simulink model "newmodel"  (R2020b)
settings: Solver=VariableStepAuto  StartTime=0.0  StopTime=10.0  RelTol=1e-3
settings Model: Creator=Obian  LastModifiedBy=Obian

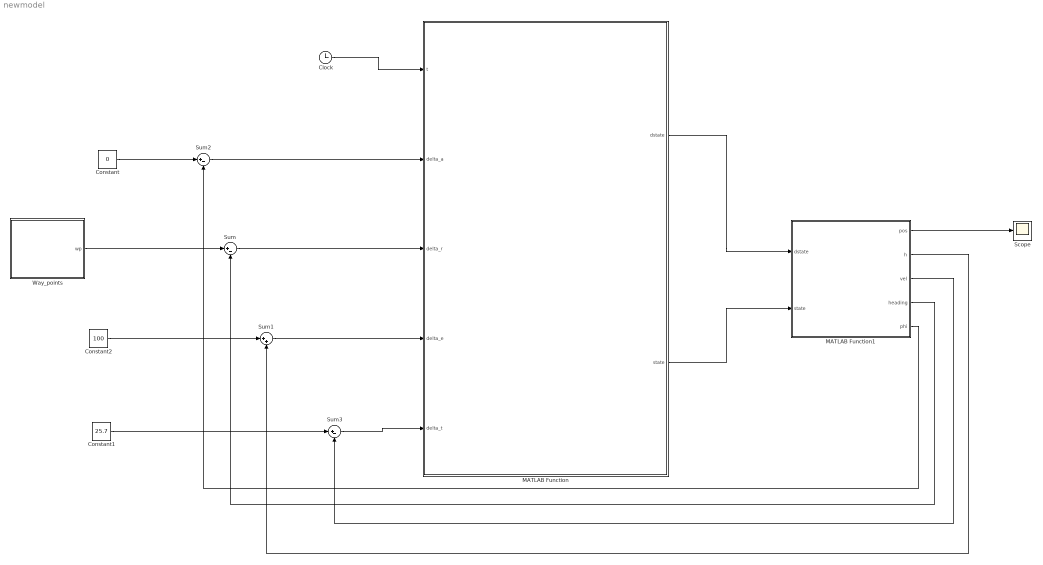
== system newmodel ==
  Clock : Clock
  Constant : Constant  Value=0
  Constant1 : Constant  Value=25.7
  Constant2 : Constant  Value=100
  MATLAB Function : MATLAB Function  TreatAsAtomicUnit=on
  MATLAB Function1 : MATLAB Function  TreatAsAtomicUnit=on
  Scope : Scope
  Sum : Sum  Inputs=|+-
  Sum1 : Sum  Inputs=|++
  Sum2 : Sum  Inputs=|+-
  Sum3 : Sum  Inputs=|+-
  Way_points : MATLAB Function  TreatAsAtomicUnit=on
  wires:
  Clock/1 -> MATLAB Function/1(t)
  MATLAB Function/1(dstate) -> MATLAB Function1/1(dstate)
  Sum/1 -> MATLAB Function/3(delta_r)
  MATLAB Function1/4(heading) -> Sum/2
  Sum1/1 -> MATLAB Function/4(delta_e)
  MATLAB Function1/2(h) -> Sum1/2
  Sum2/1 -> MATLAB Function/2(delta_a)
  Constant/1 -> Sum2/1
  Sum3/1 -> MATLAB Function/5(delta_t)
  MATLAB Function1/3(vel) -> Sum3/2
  Constant1/1 -> Sum3/1
  MATLAB Function1/5(phi) -> Sum2/2
  Constant2/1 -> Sum1/1
  MATLAB Function/2(state) -> MATLAB Function1/2(state)
  MATLAB Function1/1(pos) -> Scope/1
  Way_points/1(wp) -> Sum/1

== matlab function newmodel/MATLAB Function1 ==
  data: dstate input; pos output; h output; state input; vel output; heading output; phi output
function [pos, h, vel, heading, phi] = fcn(dstate, state)

dt = 0.1;
new_state = state + dstate.*dt;

h = new_state(3);
vel = norm(new_state(4:6));
pos = new_state(1:2);
heading = atan(new_state(2)/new_state(1));
phi = new_state(7);

return

== matlab function newmodel/MATLAB Function ==
  data: t input; delta_a input; delta_r input; delta_e input; delta_t input; dstate output; state output
function [dstate, state]  = fcn(t, delta_a, delta_r, delta_e, delta_t)

P = uav1(alpha);

Va = 27.3; %airspeed, m/s

% constants
g = 9.80665; % gravitational acceleration, P.mass/s^2
rho =  1.2133;  %kg/P.mass^3, density of air at 100 P.mass height (assume to be constant)
% alpha=0;

beta = 0.1;

% psi=0;

state = [0, 0, 100, 22.4, 15.2, 3.8, 0, 0, 0, 0, 0, 0];

n = state(1);
e = state(2);
h = state(3);
u = state(4);
v = state(5);
w = state(6);
phi = state(7);
theta = state(8);
psi = state(9);
p = state(10);
q = state(11);
r = state(12);



%% LATERAL state-space, x = [v p r phi, psi]
Yv = (rho*P.S_wing*P.b*v/(4*P.mass*Va))*(P.C_Y_p*p + P.C_Y_r*r) ...
    + (rho*P.S_wing*v/P.mass)*(P.C_Y_0+P.C_Y_beta*beta*+P.C_Y_delta_a*delta_a+P.C_Y_delta_r*delta_r)...
    + (rho*P.S_wing*P.C_Y_beta/(2*P.mass))*norm([u, w]);
Yp = w + (rho*Va*P.S_wing*P.b/(4*P.mass))*P.C_Y_p;
Yr = -u + (rho*Va*P.S_wing*P.b/(4*P.mass))*P.C_Y_r;
Yda = (rho*Va^2*P.S_wing/(2*P.mass))*P.C_Y_delta_a;
Ydr = (rho*Va^2*P.S_wing/(2*P.mass))*P.C_Y_delta_r;

Lv = (rho*P.S_wing*P.b^2*v/(4*Va))*(P.C_p_p*p + P.C_p_r*r) ...
    + (rho*P.S_wing*P.b*v)*(P.C_p_0+P.C_p_beta*beta+P.C_p_delta_a*delta_a+P.C_p_delta_r*delta_r)...
    + (rho*P.S_wing*P.b*P.C_p_beta/2)*norm([u, w]);
Lp = P.Gamma_1*q + (rho*Va*P.S_wing*P.b^2/4)*P.C_p_p;
Lr = -P.Gamma_2*q + (rho*Va*P.S_wing*P.b^2/4)*P.C_p_r;
Lda = (rho*Va^2*P.S_wing*P.b/2)*P.C_p_delta_a;
Ldr = (rho*Va^2*P.S_wing*P.b/2)*P.C_p_delta_r;

Nv = (rho*P.S_wing*P.b^2*v/(4*Va))*(P.C_r_p*p + P.C_r_r*r) ...
    + (rho*P.S_wing*P.b*v)*(P.C_r_0+P.C_r_beta*beta+P.C_r_delta_a*delta_a+P.C_r_delta_r*delta_r)...
    + (rho*P.S_wing*P.b*P.C_r_beta)*norm([u, w]);
Np = P.Gamma_7*q + (rho*Va*P.S_wing*P.b^2/4)*P.C_r_p;
Nr = -P.Gamma_1*q + (rho*Va*P.S_wing*P.b^2/4)*P.C_r_r;
Nda = (rho*Va^2*P.S_wing*P.b/2)*P.C_r_delta_a;
Ndr = (rho*Va^2*P.S_wing*P.b/2)*P.C_r_delta_r;


%% LONGITUDINAL state space, x = [u w q theta h]
Xu = (u*rho*P.S_wing/P.mass)*(P.C_X_0+(0.1)*P.C_X_alpha+P.C_X_delta_e*delta_e) - (rho*P.S_wing*w*P.C_X_alpha/(2*P.mass)) ...
    + (rho*P.S_wing*P.c*P.C_X_q*u*q/(4*P.mass*Va)); %- (rho*Sprop*Cprop*u/P.mass); 
Xw = -q +  (w*rho*P.S_wing/P.mass)*(P.C_X_0+(0.1)*P.C_X_alpha+P.C_X_delta_e*delta_e) + (rho*P.S_wing*u*P.C_X_alpha/(2*P.mass)) ...
    + (rho*P.S_wing*P.c*P.C_X_q*w*q/(4*P.mass*Va)); %(rho*Sprop*Cprop*w/P.mass); 
Xq = -w + (rho*Va*P.S_wing*P.C_X_q*P.c)/(4*P.mass);
Xde = (rho*Va^2*P.S_wing*P.C_X_delta_e)/(2*P.mass);
% Xdt = rho*Sprop*Cprop*k^2*delta_t/P.mass;
Xdt = P.F_prop/P.mass;

Zu = q +  (u*rho*P.S_wing/P.mass)*(P.C_Z_0+P.C_Z_alpha*(0.1)+P.C_Z_delta_e*delta_e) - (rho*P.S_wing*w*P.C_Z_alpha/(2*P.mass)) ...
    + (u*rho*P.S_wing*P.c*P.C_Z_q*q/(4*P.mass*Va)); 
Zw = (w*rho*P.S_wing/P.mass)*(P.C_Z_0+(0.1)*P.C_Z_alpha+P.C_Z_delta_e*delta_e) + (rho*P.S_wing*u*P.C_Z_alpha/(2*P.mass)) ...
    + (w*rho*P.S_wing*P.c*P.C_Z_q*q/(4*P.mass*Va));  
Zq = u + (rho*Va*P.S_wing*P.C_X_q*P.c)/(4*P.mass);
Zde = (rho*Va^2*P.S_wing*P.C_X_delta_e)/(2*P.mass);

Mu = (u*rho*P.S_wing*P.c/P.Jy)*(P.C_m_0+(0.1)*P.C_m_alpha+P.C_m_delta_e*delta_e) - (rho*P.S_wing*P.c*P.C_m_alpha*w)/(2*P.Jy) ...
    + (rho*P.S_wing*P.c^2*P.C_m_q*q*u)/(4*P.Jy*Va);
Mw = (w*rho*P.S_wing*P.c/P.Jy)*(P.C_m_0+(0.1)*P.C_m_alpha+P.C_m_delta_e*delta_e) + (rho*P.S_wing*P.c*P.C_m_alpha*u)/(2*P.Jy) ...
    + (rho*P.S_wing*P.c^2*P.C_m_q*q*w)/(4*P.Jy*Va);
Mq = (rho*Va*P.S_wing*P.c^2*P.C_m_q)/(4*P.Jy);
Mde = (rho*Va^2*P.S_wing*P.c*P.C_m_delta_e)/(4*P.Jy);


theta_star = theta - 0.60269;
phi_star = phi - 1.161;
% q_star = q;
% p_star = p;
% r = r;
u_star = u - 22.4175;
w_star = w - 3.7501;

        % Lateral space model
        
        dv=Yv*v+Yp*p+Yr*r+g*cos(theta_star)*cos(phi_star)*phi+Yda*delta_a+Ydr*delta_r;
        dp=Lv*v+Lp*p+Lr*r+Lda*delta_a+Ldr*delta_r;
        dr=Nv*v+Np*p+Nr*r+Nda*delta_a+Ndr*delta_r;
        dphi=p+cos(phi_star)*tan(theta_star)*r*sin(phi_star)*tan(theta_star);
        dpsi=cos(phi_star)*sec(theta_star)*r+p*cos(phi_star)*sec(theta_star)*phi;

   

        % Longitudinal space model

        du = Xu*u + Xw*w + Xq*q -g*cos(theta_star)*theta + Xde*delta_e + Xdt*delta_t;
        dw = Zu*u + Zw*w + Zq*q -g*sin(theta_star)*theta + Zde*delta_e;
        dq = Mu*u + Mw*w + Mq*q + Mde*delta_e;
        dtheta = q;
        dh = sin(theta_star)*u -cos(theta_star)*w + (u_star*cos(theta_star)+w_star*sin(theta_star))*theta;

        % n, e, h from euler transformation
        
        dn = u*cos(theta)*cos(psi) + v*(sin(phi)*sin(theta)*cos(psi) - cos(phi)*sin(psi)) + w*(cos(phi)*sin(theta)*cos(psi) + sin(phi)*sin(psi));
        de = u*cos(theta)*sin(psi) + v*(sin(phi)*sin(theta)*sin(psi) + cos(phi)*cos(psi)) + w*(cos(phi)*sin(theta)*sin(psi) - sin(phi)*cos(psi));
% % %         dh = -u*sin(theta) + v*sin(phi)*cos(theta) + w*cos(phi)*cos(theta);  % h = -pz



% n = state(1);
% e = state(2);
% h = state(3);
% u = state(4);
% v = state(5);
% w = state(6);
% phi = state(7);
% theta = state(8);
% psi = state(9);
% p = state(10);
% q = state(11);
% r = state(12);       



dstate = [dn, de, dh, du, dv, dw, dphi, dtheta, dpsi, dp, dq, dr];
        
% % dstate(1) = dn;
% % dstate(2) = de;
% % dstate(3) = dh;
% % dstate(4) = du;
% % dstate(5) = dv;
% % dstate(6) = dw;
% % dstate(7) = dphi;
% % dstate(8) = dtheta;
% % dstate(9) = dpsi;
% % dstate(10) = dp;
% % dstate(11) = dq;
% % dstate(12) = dr;

return

== matlab function newmodel/Way_points ==
  data: wp output

function wp = find_waypoints
%{
ME528 Group Assignment Waypoint Generator

Function that generates 5 waypoints. The waypoints are randomly generated
within certain limits each time the function is called. 
The UAV will start at the first waypoint (given by wp(1,1:3)) and must pass
each subsequent waypoint in order from row 1 to row 5. The UAV must pass 
within a distance of 1 m of each waypoint. The first waypoint will always
be (0,0,100) m. 

INPUTS: none

OUTPUTS:
wp = matrix of waypoints, where wp(i,1:3) are the x,y,z coordinates of the ith
waypoint in the inertial reference frame. The z-coordinate is height,
relative to the ground. All coordinates are given in metres. 
%}

rng('shuffle');

% initialise matrix to starting point of the UAV
wp = meshgrid([0 0 100], 1:5);

% Second waypoint
wp(2,1) = 500 + rand(1)*100;
wp(2,2) = wp(2,1)*tan(pi/6 + rand(1)*0.2);

% Third waypoint
dy3 = 800 + rand(1)*200;
an3 = deg2rad(70) +  rand(1)*deg2rad(15);
dx3 =1000*cos(an3);
wp(3,1:2) = [wp(2,1)-dx3, wp(2,2)+dy3];

% Fourth waypoint
dx4 = 1800 + rand(1)*500;
an4 = deg2rad(10) +  rand(1)*deg2rad(15);
dy4 = 1000*sin(an4);
wp(4,1:2) = [wp(3,1)+dx4, wp(3,2)+dy4];

% Fifth and last waypoint
dx5 = 100 - rand(1)*20;
an5 = deg2rad(15) - rand(1)*deg2rad(30);
dy5 = (1000 + rand(1)*500)*cos(an5);
wp(5,1:2) = [wp(4,1)+dx5, wp(4,2)+dy5];

return
